simulink model "AGUILAR_ARTURO_PRACTICA6"  (R2018a)
settings: Solver=VariableStepAuto  StartTime=0.0  StopTime=2  RelTol=1e-3
InitFcn:
  | M=2
  | m=0.1
  | l=0.5
  | g=9.81
  | 
  | f=1
settings Model: Creator=Arturo  LastModifiedBy=Arturo

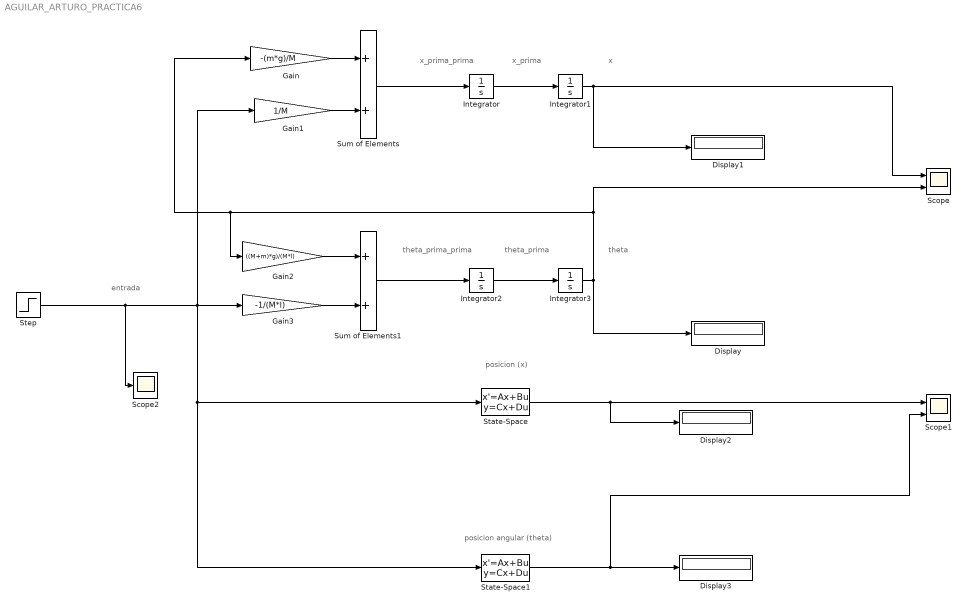
== system AGUILAR_ARTURO_PRACTICA6 ==
  note: posicion angular (theta)
  note: posicion (x)
  note: entrada
  note: theta
  note: x
  note: x_prima
  note: x_prima_prima
  note: theta_prima
  note: theta_prima_prima
  Display{,1..3} (4 alike) : Display
  Gain : Gain  Gain=-(m*g)/M
  Gain1 : Gain  Gain=1/M
  Gain2 : Gain  Gain=((M+m)*g)/(M*l)
  Gain3 : Gain  Gain=-1/(M*l)
  Integrator{,1..3} (4 alike) : Integrator
  Scope : Scope  NumInputPorts=2
  Scope1 : Scope  NumInputPorts=2
  Scope2 : Scope
  State-Space : StateSpace  A=[0 1 0 0;((M+m)*g)/(M*l) 0 0 0; 0 0 0 1;-(m*g)/M 0 0 0]  B=[0; -1/(M*l); 0; 1/M]  C=[0 0 1 0]  D=0  InitialCondition=[0 0 0 0]
  State-Space1 : StateSpace  A=[0 1 0 0;((M+m)*g)/(M*l) 0 0 0; 0 0 0 1;-(m*g)/M 0 0 0]  B=[0; -1/(M*l); 0; 1/M]  C=[1 0 0 0]  D=0  InitialCondition=[0 0 0 0]
  Step : Step  Time=0  SampleTime=0
  Sum of Elements : Sum  Inputs=2
  Sum of Elements1 : Sum  Inputs=2
  wires:
  Integrator/1 -> Integrator1/1
  Integrator2/1 -> Integrator3/1
  Gain/1 -> Sum of Elements/1
  Gain1/1 -> Sum of Elements/2
  Sum of Elements/1 -> Integrator/1
  Gain2/1 -> Sum of Elements1/1
  Sum of Elements1/1 -> Integrator2/1
  Integrator3/1 -> Display/1, Scope/2, Gain/1, Gain2/1
  Gain3/1 -> Sum of Elements1/2
  Step/1 -> Scope2/1, State-Space1/1, State-Space/1, Gain1/1, Gain3/1
  State-Space1/1 -> Scope1/2, Display3/1
  Integrator1/1 -> Display1/1, Scope/1
  State-Space/1 -> Display2/1, Scope1/1
